simulink model "voxel_cloud_node_debag"  (R2021b)
settings: Solver=FixedStepAuto  StartTime=0.0  StopTime=10.0  RelTol=1e-3
model workspace (MAT data in the model file):
  Logfile_Data_Object = ros2bag
  Logfile_Data_Object.FilePath = 'C:\Users\takumi onozawa\Documents\MATLAB\ros2bag\lidars_point_raw_0.db3'
  Logfile_Data_Object.StartTime = 1633675920681641206
  Logfile_Data_Object.EndTime = 1633676017682751873
  Logfile_Data_Object.AvailableTopics = table
  Logfile_Data_Object.AvailableTopics.data{1} = [969; 970]
  Logfile_Data_Object.AvailableTopics.data{2} = categorical
  Logfile_Data_Object.AvailableTopics.data{2}.categoryNames = {'sensor_msgs/PointCloud2'}
  Logfile_Data_Object.AvailableTopics.data{2}.codes = [1; 1]
  Logfile_Data_Object.AvailableTopics.data{3}{1} = '% contain additional information such as normals, intensity, etc. The
    | % point data is stored as a binary blob, its layout described by the
    | % contents of the "fields" array.
    | %
    | % The point cloud data may be organized 2d (image-like) or 1d (unordered).
    | % Point clouds organized as 2d images may be produced by camera depth sensors
    | % such as stereo or Time-of-flight.
    | 
    | % Time of sensor data acquisition, and the coordinate frame ID (for 3d points).
    | std_msgs/Header header
    | 
    | % 2D structure of the point cloud. If the cloud is unordered, height is
    | % 1 and width is the length of the point cloud.
    | uint32 height
    | uint32 width
    | 
    | % Describes the channels and their layout in the binary data blob.
    | PointField[] fields
    | 
    | logical    is_bigendian % Is this data bigendian?
    | uint32  point_step      % Length of a point in bytes
    | uint32  row_step        % Length of a row in bytes
    | uint8[] data            % Actual point data, size is (row_step*height)
    | 
    | logical is_dense        % True if there are no invalid points'
  Logfile_Data_Object.AvailableTopics.data{3}{2} = '% contain additional information such as normals, intensity, etc. The
    | % point data is stored as a binary blob, its layout described by the
    | % contents of the "fields" array.
    | %
    | % The point cloud data may be organized 2d (image-like) or 1d (unordered).
    | % Point clouds organized as 2d images may be produced by camera depth sensors
    | % such as stereo or Time-of-flight.
    | 
    | % Time of sensor data acquisition, and the coordinate frame ID (for 3d points).
    | std_msgs/Header header
    | 
    | % 2D structure of the point cloud. If the cloud is unordered, height is
    | % 1 and width is the length of the point cloud.
    | uint32 height
    | uint32 width
    | 
    | % Describes the channels and their layout in the binary data blob.
    | PointField[] fields
    | 
    | logical    is_bigendian % Is this data bigendian?
    | uint32  point_step      % Length of a point in bytes
    | uint32  row_step        % Length of a row in bytes
    | uint8[] data            % Actual point data, size is (row_step*height)
    | 
    | logical is_dense        % True if there are no invalid points'
  Logfile_Data_Object.AvailableTopics.ndims = 2
  Logfile_Data_Object.AvailableTopics.nrows = 2
  Logfile_Data_Object.AvailableTopics.rownames = {'/lidar_front/points_raw'; '/lidar_rear/points_raw'}
  Logfile_Data_Object.AvailableTopics.nvars = 3
  Logfile_Data_Object.AvailableTopics.varnames = {'NumMessages', 'MessageType', 'MessageDefinition'}
  Logfile_Data_Object.AvailableTopics.props.useVariableNamesOriginal = 0
  Logfile_Data_Object.AvailableTopics.props.useDimensionNamesOriginal = 0
  Logfile_Data_Object.AvailableTopics.props.CustomProps = struct()
  Logfile_Data_Object.AvailableTopics.props.VariableCustomProps = struct()
  Logfile_Data_Object.AvailableTopics.props.versionSavedFrom = 4
  Logfile_Data_Object.AvailableTopics.props.minCompatibleVersion = 1
  Logfile_Data_Object.AvailableTopics.props.incompatibilityMsg = ''
  Logfile_Data_Object.AvailableTopics.props.VersionSavedFrom = 4
  Logfile_Data_Object.AvailableTopics.props.Description = ''
  Logfile_Data_Object.AvailableTopics.props.VariableNamesOriginal = {}
  Logfile_Data_Object.AvailableTopics.props.DimensionNames = {'Row', 'Variables'}
  Logfile_Data_Object.AvailableTopics.props.DimensionNamesOriginal = {}
  Logfile_Data_Object.AvailableTopics.props.UserData = []
  Logfile_Data_Object.AvailableTopics.props.VariableDescriptions = {}
  Logfile_Data_Object.AvailableTopics.props.VariableUnits = {}
  Logfile_Data_Object.AvailableTopics.props.VariableContinuity = {}
  Logfile_Data_Object.MessageList = table
  Logfile_Data_Object.MessageList.data{1} = [1633675920681641206 1633675920704850047 1633675920710280571 1633675920841302537 1633675920849007917 1633675920944718285 1633675920950454411 1633675921046456357 1633675921051238695 1633675921143527086 1633675921154682295 1633675921262758351 ... (1939 elements, 1939x1)]
  Logfile_Data_Object.MessageList.data{2} = categorical
  Logfile_Data_Object.MessageList.data{2}.categoryNames = {'/lidar_rear/points_raw'; '/lidar_front/points_raw'}
  Logfile_Data_Object.MessageList.data{2}.codes = [1 2 1 2 1 2 1 2 1 2 1 2 ... (1939 elements, 1939x1)]
  Logfile_Data_Object.MessageList.data{3} = categorical
  Logfile_Data_Object.MessageList.data{3}.categoryNames = {'sensor_msgs/PointCloud2'}
  Logfile_Data_Object.MessageList.data{3}.codes = [1 1 1 1 1 1 1 1 1 1 1 1 ... (1939 elements, 1939x1)]
  Logfile_Data_Object.MessageList.ndims = 2
  Logfile_Data_Object.MessageList.nrows = 1939
  Logfile_Data_Object.MessageList.nvars = 3
  Logfile_Data_Object.MessageList.varnames = {'Time', 'Topic', 'MessageType'}
  Logfile_Data_Object.MessageList.props.useVariableNamesOriginal = 0
  Logfile_Data_Object.MessageList.props.useDimensionNamesOriginal = 0
  Logfile_Data_Object.MessageList.props.CustomProps = struct()
  Logfile_Data_Object.MessageList.props.VariableCustomProps = struct()
  Logfile_Data_Object.MessageList.props.versionSavedFrom = 4
  Logfile_Data_Object.MessageList.props.minCompatibleVersion = 1
  Logfile_Data_Object.MessageList.props.incompatibilityMsg = ''
  Logfile_Data_Object.MessageList.props.VersionSavedFrom = 4
  Logfile_Data_Object.MessageList.props.Description = ''
  Logfile_Data_Object.MessageList.props.VariableNamesOriginal = {}
  Logfile_Data_Object.MessageList.props.DimensionNames = {'Row', 'Variables'}
  Logfile_Data_Object.MessageList.props.DimensionNamesOriginal = {}
  Logfile_Data_Object.MessageList.props.UserData = []
  Logfile_Data_Object.MessageList.props.VariableDescriptions = {}
  Logfile_Data_Object.MessageList.props.VariableUnits = {}
  Logfile_Data_Object.MessageList.props.VariableContinuity = {}
  Logfile_Data_Object.TopicTypeMap = containers.Map
  Logfile_Data_Object.TopicTypeMap.serialization.keys = {'/lidar_front/points_raw', '/lidar_rear/points_raw'}
  Logfile_Data_Object.TopicTypeMap.serialization.values = {'sensor_msgs/PointCloud2', 'sensor_msgs/PointCloud2'}
  Logfile_Data_Object.TopicTypeMap.serialization.uniformity = 1
  Logfile_Data_Object.TopicTypeMap.serialization.keyType = 'char'
  Logfile_Data_Object.TopicTypeMap.serialization.valueType = 'char'
  Logfile_Data_Object.TopicDefinitionMap = containers.Map
  Logfile_Data_Object.TopicDefinitionMap.serialization.keys = {'/lidar_front/points_raw', '/lidar_rear/points_raw'}
  Logfile_Data_Object.TopicDefinitionMap.serialization.values{1} = '% contain additional information such as normals, intensity, etc. The
    | % point data is stored as a binary blob, its layout described by the
    | % contents of the "fields" array.
    | %
    | % The point cloud data may be organized 2d (image-like) or 1d (unordered).
    | % Point clouds organized as 2d images may be produced by camera depth sensors
    | % such as stereo or Time-of-flight.
    | 
    | % Time of sensor data acquisition, and the coordinate frame ID (for 3d points).
    | std_msgs/Header header
    | 
    | % 2D structure of the point cloud. If the cloud is unordered, height is
    | % 1 and width is the length of the point cloud.
    | uint32 height
    | uint32 width
    | 
    | % Describes the channels and their layout in the binary data blob.
    | PointField[] fields
    | 
    | logical    is_bigendian % Is this data bigendian?
    | uint32  point_step      % Length of a point in bytes
    | uint32  row_step        % Length of a row in bytes
    | uint8[] data            % Actual point data, size is (row_step*height)
    | 
    | logical is_dense        % True if there are no invalid points'
  Logfile_Data_Object.TopicDefinitionMap.serialization.values{2} = '% contain additional information such as normals, intensity, etc. The
    | % point data is stored as a binary blob, its layout described by the
    | % contents of the "fields" array.
    | %
    | % The point cloud data may be organized 2d (image-like) or 1d (unordered).
    | % Point clouds organized as 2d images may be produced by camera depth sensors
    | % such as stereo or Time-of-flight.
    | 
    | % Time of sensor data acquisition, and the coordinate frame ID (for 3d points).
    | std_msgs/Header header
    | 
    | % 2D structure of the point cloud. If the cloud is unordered, height is
    | % 1 and width is the length of the point cloud.
    | uint32 height
    | uint32 width
    | 
    | % Describes the channels and their layout in the binary data blob.
    | PointField[] fields
    | 
    | logical    is_bigendian % Is this data bigendian?
    | uint32  point_step      % Length of a point in bytes
    | uint32  row_step        % Length of a row in bytes
    | uint8[] data            % Actual point data, size is (row_step*height)
    | 
    | logical is_dense        % True if there are no invalid points'
  Logfile_Data_Object.TopicDefinitionMap.serialization.uniformity = 1
  Logfile_Data_Object.TopicDefinitionMap.serialization.keyType = 'char'
  Logfile_Data_Object.TopicDefinitionMap.serialization.valueType = 'char'
  Logfile_Path = 'C:\Users\takumi onozawa\Documents\MATLAB\ros2bag\lidars_point_raw_0.db3'
  Logfile_Playback_Duration = nan
  Logfile_Playback_Offset = nan
  SL_ROS_VariableLengthArrays_MaxSizes.CommonInfo.ArrayTruncateAction = 'EmitWarning'
  SL_ROS_VariableLengthArrays_MaxSizes.MsgTypeMap = containers.Map
  SL_ROS_VariableLengthArrays_MaxSizes.MsgTypeMap.serialization.keys = {'sensor_msgs/PointCloud2'}
  SL_ROS_VariableLengthArrays_MaxSizes.MsgTypeMap.serialization.values{1}(1).PropertyName = 'data'
  SL_ROS_VariableLengthArrays_MaxSizes.MsgTypeMap.serialization.values{1}(1).DataType = 'uint8'
  SL_ROS_VariableLengthArrays_MaxSizes.MsgTypeMap.serialization.values{1}(1).MaxLength = 1760000
  SL_ROS_VariableLengthArrays_MaxSizes.MsgTypeMap.serialization.values{1}(2).PropertyName = 'fields'
  SL_ROS_VariableLengthArrays_MaxSizes.MsgTypeMap.serialization.values{1}(2).DataType = 'sensor_msgs/PointField'
  SL_ROS_VariableLengthArrays_MaxSizes.MsgTypeMap.serialization.values{1}(2).MaxLength = 16
  SL_ROS_VariableLengthArrays_MaxSizes.MsgTypeMap.serialization.uniformity = 0
  SL_ROS_VariableLengthArrays_MaxSizes.MsgTypeMap.serialization.keyType = 'char'
  SL_ROS_VariableLengthArrays_MaxSizes.MsgTypeMap.serialization.valueType = 'any'
undefined symbols (not defined in the file or in its folder): height, row_step, width
libraries: ros2lib x4, simulink x4
settings Model: Creator=takum  LastModifiedBy=takumi onozawa
settings SolverCC: AlgebraicLoopSolver=TrustRegion
settings OptimizationCC: EnhancedBackFolding=on  PassReuseOutputArgsAs=Individual arguments  ZeroExternalMemoryAtStartup=off  ZeroInternalMemoryAtStartup=off  MaxStackSize=64  OptimizeBlockOrder=speed  DifferentSizesBufferReuse=on  OptimizationCustomize=off  EfficientTunableParamExpr=on
settings DebuggingCC: ParameterTunabilityLossMsg=error  SFMachineParentedDataDiag=warning
settings SFSimCC: MATLABDynamicMemAlloc=off
settings RTWCC: Description=Embedded Coder  SystemTargetFile=ert.tlc  HardwareBoard=Robot Operating System 2 (ROS 2)  TemplateMakefile=ert_default_tmf  Toolchain=Colcon Tools  TargetLang=C++
settings CodeAppCC: ForceParamTrailComments=on  IgnoreCustomStorageClasses=off  OperatorAnnotations=on  SimulinkDataObjDesc=on  SFDataObjDesc=on  InsertBlockDesc=on
settings ERTTargetCC: CodeInterfacePackaging=C++ class  RootIOFormat=Structure reference

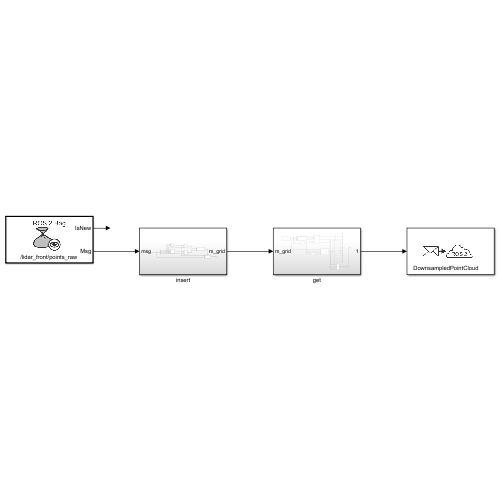
[thumbnail: Simulink's stored preview of the top-level diagram]
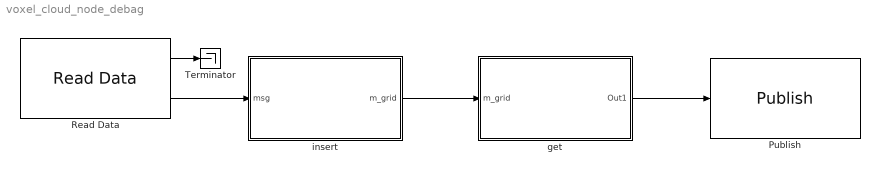
== system voxel_cloud_node_debag ==
  Publish : ros2lib/Publish  topicSource=Specify your own  topic=DownsampledPointCloud  messageType=sensor_msgs/PointCloud2  QOSHistory=Keep last  QOSDepth=1  QOSReliability=Reliable  QOSDurability=Volatile
      settings: SourceProductBaseCode=RR
  Read Data : ros2lib/Read Data  topic=/lidar_front/points_raw  sampleTime=-1  logfileType=rosbag2  modelName=voxel_cloud_node_debag  msgType=sensor_msgs/PointCloud2
      settings: SourceProductBaseCode=RR
  Terminator : Terminator
  get : Subsystem
  insert : Subsystem
  wires:
  Read Data/1 -> Terminator/1
  Read Data/2 -> insert/1(msg)
  get/1(Out1) -> Publish/1
  insert/1(m_grid) -> get/1(m_grid)

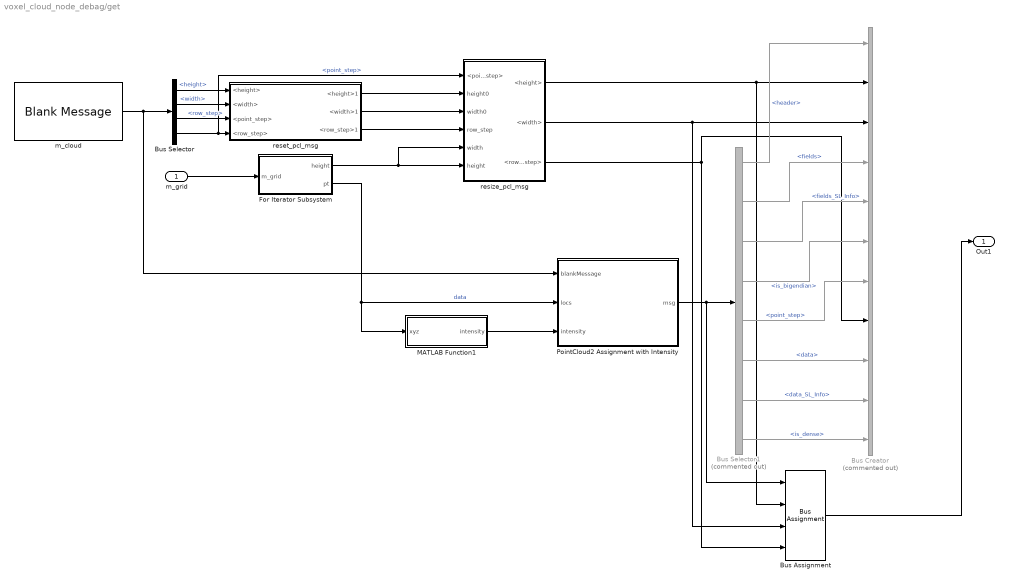
== system voxel_cloud_node_debag/get ==
  m_grid : Inport
  Bus Assignment : BusAssignment  AssignedSignals=height,width,row_step
  Bus Creator : BusCreator  Commented=on  Inputs=11
  Bus Selector : BusSelector  OutputSignals=height,width,row_step,point_step
  Bus Selector1 : BusSelector  Commented=on  OutputSignals=header,fields,fields_SL_Info,is_bigendian,point_step,data,data_SL_Info,is_dense
  For Iterator Subsystem : Subsystem  TreatAsAtomicUnit=on
  MATLAB Function1 : MATLAB Function  TreatAsAtomicUnit=on
  PointCloud2 Assignment with Intensity : MATLAB Function  TreatAsAtomicUnit=on
  m_cloud : ros2lib/Blank Message  messageClass=Message  entityType=sensor_msgs/PointCloud2  messageType=sensor_msgs/PointCloud2  SampleTime=inf
      settings: SourceProductBaseCode=RR
  reset_pcl_msg : Subsystem
  resize_pcl_msg : Subsystem
  Out1 : Outport
  wires:
  m_grid/1 -> For Iterator Subsystem/1(m_grid)
  Bus Selector/2 -> reset_pcl_msg/2(<width>)  "<width>"
  Bus Selector/3 -> reset_pcl_msg/3(<point_step>)  "<row_step>"
  Bus Selector/1 -> reset_pcl_msg/1(<height>)  "<height>"
  For Iterator Subsystem/2(pt) -> PointCloud2 Assignment with Intensity/2(locs), MATLAB Function1/1(xyz)  "data"
  Bus Selector/4 -> resize_pcl_msg/1(<point_step>), reset_pcl_msg/4(<row_step>)  "<point_step>"
  resize_pcl_msg/3(<row_step>) -> Bus Creator/8, Bus Assignment/4
  resize_pcl_msg/2(<width>) -> Bus Assignment/3, Bus Creator/3
  reset_pcl_msg/1(<height>1) -> resize_pcl_msg/2(height0)
  reset_pcl_msg/3(<row_step>1) -> resize_pcl_msg/4(row_step)
  reset_pcl_msg/2(<width>1) -> resize_pcl_msg/3(width0)
  resize_pcl_msg/1(<height>) -> Bus Assignment/2, Bus Creator/2
  For Iterator Subsystem/1(height) -> resize_pcl_msg/5(width), resize_pcl_msg/6(height)
  Bus Assignment/1 -> Out1/1
  PointCloud2 Assignment with Intensity/1(msg) -> Bus Assignment/1, Bus Selector1/1
  m_cloud/1 -> PointCloud2 Assignment with Intensity/1(blankMessage), Bus Selector/1
  Bus Selector1/1 -> Bus Creator/1  "<header>"
  Bus Selector1/2 -> Bus Creator/4  "<fields>"
  Bus Selector1/3 -> Bus Creator/5  "<fields_SL_Info>"
  Bus Selector1/4 -> Bus Creator/6  "<is_bigendian>"
  Bus Selector1/5 -> Bus Creator/7  "<point_step>"
  Bus Selector1/6 -> Bus Creator/9  "<data>"
  Bus Selector1/7 -> Bus Creator/10  "<data_SL_Info>"
  Bus Selector1/8 -> Bus Creator/11  "<is_dense>"
  MATLAB Function1/1(intensity) -> PointCloud2 Assignment with Intensity/3(intensity)

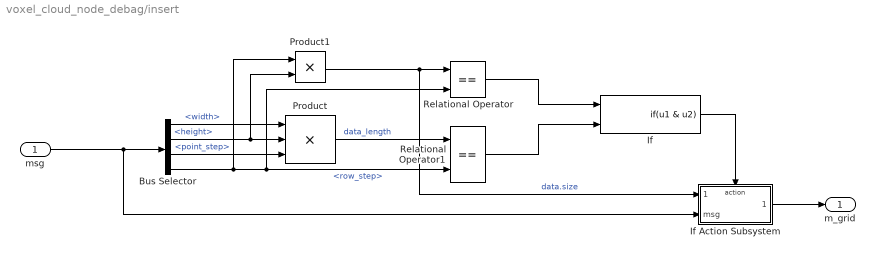
== system voxel_cloud_node_debag/insert ==
  msg : Inport
  Bus Selector : BusSelector  OutputSignals=width,height,point_step,row_step
  If : If  NumInputs=2  IfExpression=u1 & u2  ShowElse=off
  If Action Subsystem : Subsystem  TreatAsAtomicUnit=on
  Product : Product  Inputs=3
  Product1 : Product  OutDataTypeStr=uint32
  Relational Operator : RelationalOperator  Operator===  OutDataTypeStr=boolean  RndMeth=Simplest
  Relational Operator1 : RelationalOperator  Operator===  OutDataTypeStr=boolean  RndMeth=Simplest
  m_grid : Outport
  wires:
  If Action Subsystem/1(m_grid) -> m_grid/1
  Bus Selector/1 -> Product/1  "<width>"
  Bus Selector/2 -> Product/2, Product1/2  "<height>"
  Bus Selector/3 -> Product/3  "<point_step>"
  Product/1 -> Relational Operator1/1  "data_length"
  Bus Selector/4 -> Relational Operator1/2, Relational Operator/2, Product1/1  "<row_step>"
  Product1/1 -> If Action Subsystem/1(data.size), Relational Operator/1  "data.size"
  Relational Operator/1 -> If/1
  Relational Operator1/1 -> If/2
  If/1 -> If Action Subsystem/Action
  msg/1 -> Bus Selector/1, If Action Subsystem/2(msg)

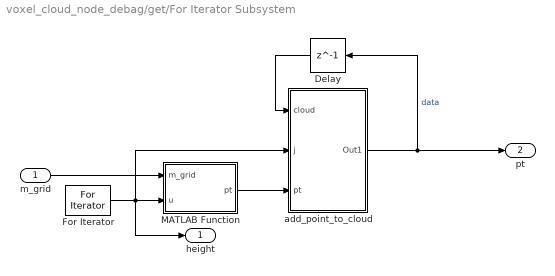
== system voxel_cloud_node_debag/get/For Iterator Subsystem ==
  m_grid : Inport
  Delay : Delay  DelayLength=1
  For Iterator : ForIterator  IterationLimit=55000
  MATLAB Function : MATLAB Function  TreatAsAtomicUnit=on
  add_point_to_cloud : Subsystem
  height : Outport
  pt : Outport  Port=2
  wires:
  m_grid/1 -> MATLAB Function/1(m_grid)
  MATLAB Function/1(pt) -> add_point_to_cloud/3(pt)
  For Iterator/1 -> height/1, add_point_to_cloud/2(j), MATLAB Function/2(u)
  add_point_to_cloud/1(Out1) -> Delay/1, pt/1  "data"
  Delay/1 -> add_point_to_cloud/1(cloud)

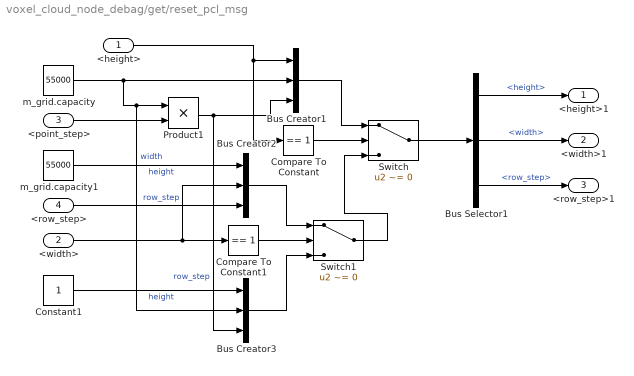
== system voxel_cloud_node_debag/get/reset_pcl_msg ==
  <height> : Inport
  <width> : Inport  Port=2
  <point_step> : Inport  Port=3
  <row_step> : Inport  Port=4
  Bus Creator1 : BusCreator  Inputs=3
  Bus Creator2 : BusCreator  Inputs=3
  Bus Creator3 : BusCreator  Inputs=3
  Bus Selector1 : BusSelector  OutputSignals=height,width,row_step
  Compare To Constant : simulink/Logic and Bit Operations/Compare To Constant  relop===  const=1  OutDataTypeStr=boolean
  Compare To Constant1 : simulink/Logic and Bit Operations/Compare To Constant  relop===  const=1  OutDataTypeStr=boolean
  Constant1 : Constant  OutDataTypeStr=uint32
  Product1 : Product  OutDataTypeStr=uint32
  Switch : Switch  Criteria=u2 ~= 0
  Switch1 : Switch  Criteria=u2 ~= 0
  m_grid.capacity : Constant  Value=55000  OutDataTypeStr=uint32
  m_grid.capacity1 : Constant  Value=55000  OutDataTypeStr=uint32
  <height>1 : Outport
  <width>1 : Outport  Port=2
  <row_step>1 : Outport  Port=3
  wires:
  <point_step>/1 -> Product1/2
  m_grid.capacity/1 -> Product1/1, Bus Creator3/2, Bus Creator1/2  "width"
  Switch/1 -> Bus Selector1/1
  Product1/1 -> Bus Creator1/3, Bus Creator3/3  "row_step"
  m_grid.capacity1/1 -> Bus Creator2/1  "height"
  Bus Creator2/1 -> Switch1/1
  Bus Creator1/1 -> Switch/1
  <height>/1 -> Compare To Constant/1, Bus Creator1/1
  Constant1/1 -> Bus Creator3/1  "height"
  Bus Creator3/1 -> Switch1/3
  Compare To Constant1/1 -> Switch1/2
  Switch1/1 -> Switch/3
  <width>/1 -> Bus Creator2/2, Compare To Constant1/1
  Compare To Constant/1 -> Switch/2
  Bus Selector1/1 -> <height>1/1  "<height>"
  <row_step>/1 -> Bus Creator2/3  "row_step"
  Bus Selector1/2 -> <width>1/1  "<width>"
  Bus Selector1/3 -> <row_step>1/1  "<row_step>"

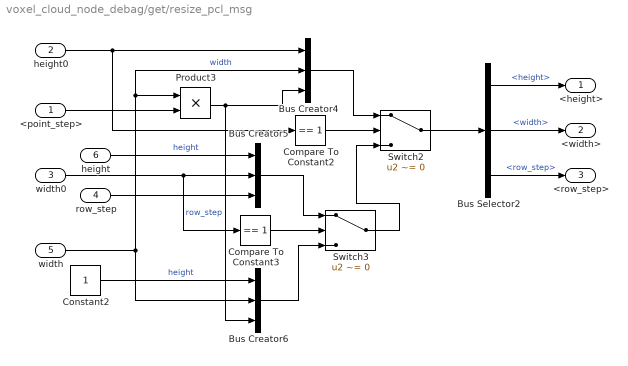
== system voxel_cloud_node_debag/get/resize_pcl_msg ==
  <point_step> : Inport
  height0 : Inport  Port=2
  width0 : Inport  Port=3
  row_step : Inport  Port=4
  width : Inport  Port=5
  height : Inport  Port=6
  Bus Creator4 : BusCreator  Inputs=3
  Bus Creator5 : BusCreator  Inputs=3
  Bus Creator6 : BusCreator  Inputs=3
  Bus Selector2 : BusSelector  OutputSignals=height,width,row_step
  Compare To Constant2 : simulink/Logic and Bit Operations/Compare To Constant  relop===  const=1  OutDataTypeStr=boolean
  Compare To Constant3 : simulink/Logic and Bit Operations/Compare To Constant  relop===  const=1  OutDataTypeStr=boolean
  Constant2 : Constant  OutDataTypeStr=uint32
  Product3 : Product  OutDataTypeStr=uint32
  Switch2 : Switch  Criteria=u2 ~= 0
  Switch3 : Switch  Criteria=u2 ~= 0
  <height> : Outport
  <width> : Outport  Port=2
  <row_step> : Outport  Port=3
  wires:
  Compare To Constant3/1 -> Switch3/2
  Bus Creator6/1 -> Switch3/3
  Switch2/1 -> Bus Selector2/1
  Product3/1 -> Bus Creator4/3, Bus Creator6/3  "row_step"
  Switch3/1 -> Switch2/3
  Bus Selector2/1 -> <height>/1  "<height>"
  width/1 -> Bus Creator6/2, Bus Creator4/2, Product3/1  "width"
  Bus Creator5/1 -> Switch3/1
  Constant2/1 -> Bus Creator6/1  "height"
  Bus Creator4/1 -> Switch2/1
  Compare To Constant2/1 -> Switch2/2
  height0/1 -> Compare To Constant2/1, Bus Creator4/1
  width0/1 -> Compare To Constant3/1, Bus Creator5/2
  Bus Selector2/3 -> <row_step>/1  "<row_step>"
  <point_step>/1 -> Product3/2
  row_step/1 -> Bus Creator5/3
  Bus Selector2/2 -> <width>/1  "<width>"
  height/1 -> Bus Creator5/1  "height"

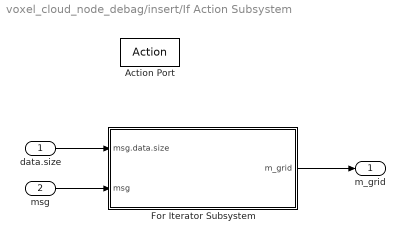
== system voxel_cloud_node_debag/insert/If Action Subsystem ==
  data.size : Inport
  msg : Inport  Port=2
  Action Port : ActionPort  ActionPortLabel=if(u1 & u2)
  For Iterator Subsystem : Subsystem  TreatAsAtomicUnit=on
  m_grid : Outport
  wires:
  data.size/1 -> For Iterator Subsystem/1(msg.data.size)
  msg/1 -> For Iterator Subsystem/2(msg)
  For Iterator Subsystem/1(m_grid) -> m_grid/1

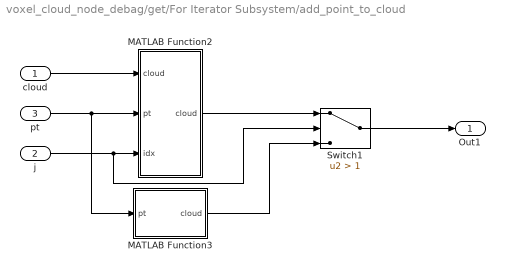
== system voxel_cloud_node_debag/get/For Iterator Subsystem/add_point_to_cloud ==
  cloud : Inport
  j : Inport  Port=2
  pt : Inport  Port=3
  MATLAB Function2 : MATLAB Function  TreatAsAtomicUnit=on
  MATLAB Function3 : MATLAB Function  TreatAsAtomicUnit=on
  Switch1 : Switch  Criteria=u2 > Threshold  Threshold=1
  Out1 : Outport
  wires:
  MATLAB Function2/1(cloud) -> Switch1/1
  pt/1 -> MATLAB Function3/1(pt), MATLAB Function2/2(pt)
  j/1 -> Switch1/2, MATLAB Function2/3(idx)
  Switch1/1 -> Out1/1
  MATLAB Function3/1(cloud) -> Switch1/3
  cloud/1 -> MATLAB Function2/1("cloud ")

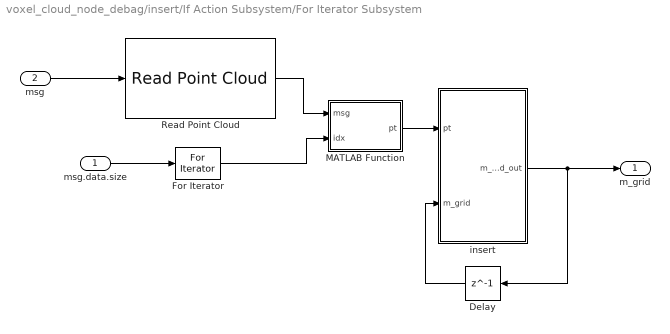
== system voxel_cloud_node_debag/insert/If Action Subsystem/For Iterator Subsystem ==
  msg.data.size : Inport
  msg : Inport  Port=2
  Delay : Delay  DelayLength=1
  For Iterator : ForIterator  IterationSource=external
  MATLAB Function : MATLAB Function  TreatAsAtomicUnit=on
  Read Point Cloud : ros2lib/Read Point Cloud  MaximumPointCloudSize=[480, 640]  PreserveStructure=off  ShowRGBOutput=off  ShowIntensityOutput=off  ShowErrorCodeOutput=off  VariableSizeOutputs=off
      settings: SourceProductBaseCode=RR
  insert : Subsystem
  m_grid : Outport
  wires:
  msg/1 -> Read Point Cloud/1
  msg.data.size/1 -> For Iterator/1
  insert/1(m_grid_out) -> Delay/1, m_grid/1
  Delay/1 -> insert/2(m_grid)
  For Iterator/1 -> MATLAB Function/2(idx)
  MATLAB Function/1(pt) -> insert/1(pt)
  Read Point Cloud/1 -> MATLAB Function/1(msg)

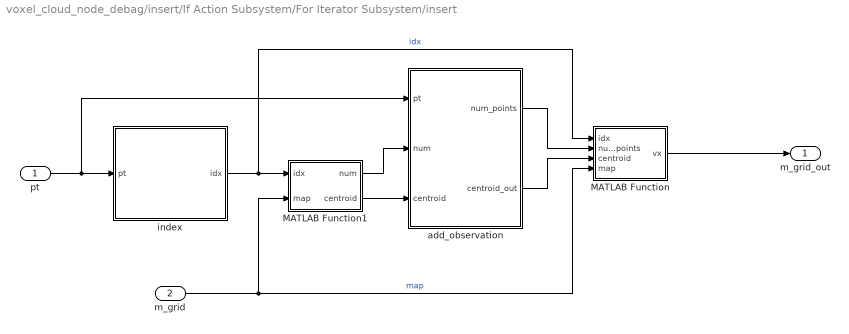
== system voxel_cloud_node_debag/insert/If Action Subsystem/For Iterator Subsystem/insert ==
  pt : Inport
  m_grid : Inport  Port=2
  MATLAB Function : MATLAB Function  TreatAsAtomicUnit=on
  MATLAB Function1 : MATLAB Function  TreatAsAtomicUnit=on
  add_observation : Subsystem
  index : Subsystem
  m_grid_out : Outport
  wires:
  pt/1 -> add_observation/1(pt), index/1(pt)
  index/1(idx) -> MATLAB Function/1(idx), MATLAB Function1/1(idx)  "idx"
  m_grid/1 -> MATLAB Function/4(map), MATLAB Function1/2(map)  "map"
  MATLAB Function/1(vx) -> m_grid_out/1
  MATLAB Function1/1(num) -> add_observation/2(num)
  add_observation/1(num_points) -> MATLAB Function/2(num_points)
  add_observation/2(centroid_out) -> MATLAB Function/3(centroid)
  MATLAB Function1/2(centroid) -> add_observation/3(centroid)

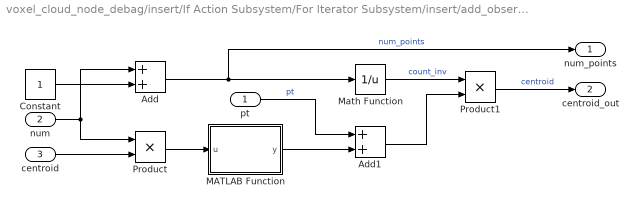
== system voxel_cloud_node_debag/insert/If Action Subsystem/For Iterator Subsystem/insert/add_observation ==
  pt : Inport
  num : Inport  Port=2
  centroid : Inport  Port=3
  Add : Sum  OutDataTypeStr=uint32
  Add1 : Sum
  Constant : Constant
  MATLAB Function : MATLAB Function  TreatAsAtomicUnit=on
  Math Function : Math  Operator=reciprocal  SaturateOnIntegerOverflow=on
  Product : Product  OutDataTypeStr=uint32
  Product1 : Product  OutDataTypeStr=double
  num_points : Outport
  centroid_out : Outport  Port=2
  wires:
  num/1 -> Product/1, Add/1
  Add/1 -> num_points/1, Math Function/1  "num_points"
  Math Function/1 -> Product1/1  "count_inv"
  Add1/1 -> Product1/2
  Product1/1 -> centroid_out/1  "centroid"
  Constant/1 -> Add/2
  Product/1 -> MATLAB Function/1(u)
  centroid/1 -> Product/2
  pt/1 -> Add1/1  "pt"
  MATLAB Function/1(y) -> Add1/2

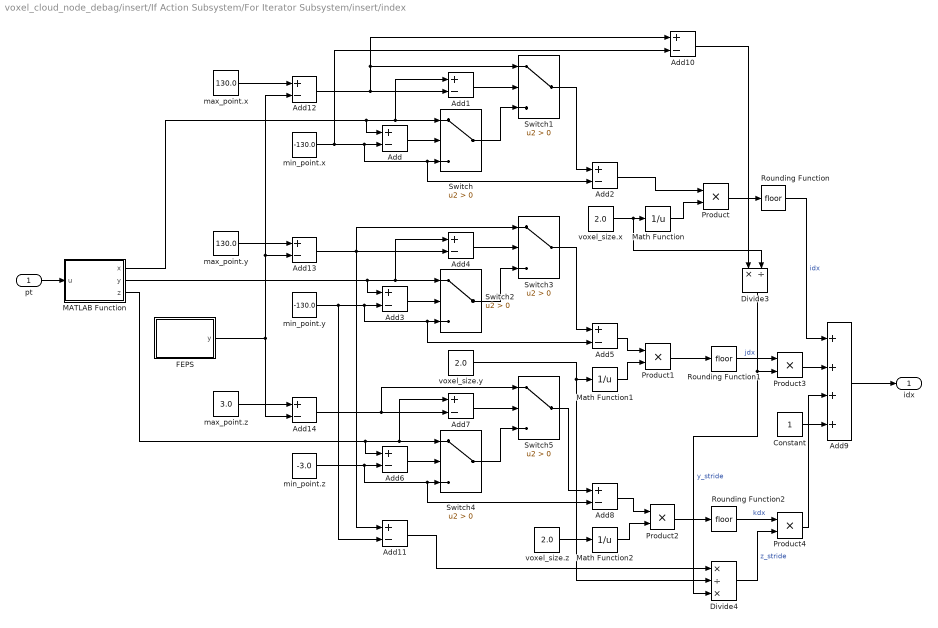
== system voxel_cloud_node_debag/insert/If Action Subsystem/For Iterator Subsystem/insert/index ==
  pt : Inport
  Add{,1..8,10..14} (14 alike) : Sum  Inputs=+-
  Add9 : Sum  Inputs=4  OutDataTypeStr=uint32
  Constant : Constant
  Divide3 : Product  Inputs=*/
  Divide4 : Product  Inputs=*/*
  FEPS : MATLAB Function  TreatAsAtomicUnit=on
  MATLAB Function : MATLAB Function  TreatAsAtomicUnit=on
  Math Function : Math  Operator=reciprocal  SaturateOnIntegerOverflow=on
  Math Function1 : Math  Operator=reciprocal  SaturateOnIntegerOverflow=on
  Math Function2 : Math  Operator=reciprocal  SaturateOnIntegerOverflow=on
  Product{,1..4} (5 alike) : Product
  Rounding Function : Rounding
  Rounding Function1 : Rounding
  Rounding Function2 : Rounding
  Switch{,1..5} (6 alike) : Switch  Criteria=u2 > Threshold
  max_point.x : Constant  Value=130.0
  max_point.y : Constant  Value=130.0
  max_point.z : Constant  Value=3.0
  min_point.x : Constant  Value=-130.0
  min_point.y : Constant  Value=-130.0
  min_point.z : Constant  Value=-3.0
  voxel_size.x : Constant  Value=2.0
  voxel_size.y : Constant  Value=2.0
  voxel_size.z : Constant  Value=2.0
  idx : Outport
  wires:
  pt/1 -> MATLAB Function/1(u)
  Add13/1 -> Switch3/1, Add4/2, Add11/1
  Math Function/1 -> Product/2
  Switch1/1 -> Add2/1
  min_point.z/1 -> Add8/2, Switch4/3, Add6/2
  Product3/1 -> Add9/2
  min_point.y/1 -> Add5/2, Switch2/3, Add3/2, Add11/2
  voxel_size.z/1 -> Math Function2/1
  Add4/1 -> Switch3/2
  Divide4/1 -> Product4/2  "z_stride"
  voxel_size.y/1 -> Math Function1/1, Divide4/2
  FEPS/1(y) -> Add14/2, Add13/2, Add12/2
  voxel_size.x/1 -> Math Function/1, Divide3/2
  Add10/1 -> Divide3/1
  Add8/1 -> Product2/1
  Product2/1 -> Rounding Function2/1
  min_point.x/1 -> Add10/2, Add2/2, Switch/3, Add/2
  Add6/1 -> Switch4/2
  Add11/1 -> Divide4/1
  Add1/1 -> Switch1/2
  Product1/1 -> Rounding Function1/1
  Divide3/1 -> Divide4/3, Product3/2  "y_stride"
  Switch4/1 -> Switch5/3
  Switch3/1 -> Add5/1
  Product/1 -> Rounding Function/1
  Switch/1 -> Switch1/3
  Add/1 -> Switch/2
  Add14/1 -> Switch5/1, Add7/2
  Add5/1 -> Product1/1
  Add12/1 -> Add1/2, Add10/1, Switch1/1
  Switch2/1 -> Switch3/3
  Add3/1 -> Switch2/2
  Math Function1/1 -> Product1/2
  Add7/1 -> Switch5/2
  Product4/1 -> Add9/3
  Add2/1 -> Product/1
  Switch5/1 -> Add8/1
  max_point.x/1 -> Add12/1
  Math Function2/1 -> Product2/2
  max_point.y/1 -> Add13/1
  max_point.z/1 -> Add14/1
  Add9/1 -> idx/1
  MATLAB Function/2(y) -> Add3/1, Add4/1, Switch2/1
  MATLAB Function/1(x) -> Add/1, Add1/1, Switch/1
  MATLAB Function/3(z) -> Add6/1, Switch4/1, Add7/1
  Rounding Function/1 -> Add9/1  "idx"
  Rounding Function1/1 -> Product3/1  "jdx"
  Rounding Function2/1 -> Product4/1  "kdx"
  Constant/1 -> Add9/4

== matlab function voxel_cloud_node_debag/get/MATLAB Function1 ==
  data: xyz input; intensity output
function intensity = fcn(xyz)
intensity = rescale(xyz(:,3),0,255);

== matlab function voxel_cloud_node_debag/insert/If Action Subsystem/For Iterator Subsystem/MATLAB Function ==
  data: pt output; msg input; idx input
function pt = fcn(msg, idx)

pt = msg(idx,:);

== matlab function voxel_cloud_node_debag/insert/If Action Subsystem/For Iterator Subsystem/insert/MATLAB Function1 ==
  data: num output; idx input; map input; centroid output
function [num,centroid] = fcn(idx, map)

num = map(idx).num;
centroid = map(idx).centroid;

== matlab function voxel_cloud_node_debag/insert/If Action Subsystem/For Iterator Subsystem/insert/MATLAB Function ==
  data: idx input; num_points input; centroid input; map input; vx output Bus: BusObject size=55000,2
function vx = fcn(idx, num_points, centroid, map)

map(idx).num = num_points;
map(idx).centroid = permute(centroid,[2 1]);
vx = map;

== matlab function voxel_cloud_node_debag/get/For Iterator Subsystem/add_point_to_cloud/MATLAB Function2 ==
  data: cloud output size=[55000 3]; cloud input; pt input; idx input
function cloud = fcn(cloud,pt, idx)
cloud(idx,:) = pt;

== matlab function voxel_cloud_node_debag/get/For Iterator Subsystem/add_point_to_cloud/MATLAB Function3 ==
  data: cloud output; pt input
function cloud = fcn(pt)
cloud = zeros(55000,3);
cloud(1,:) = pt;

== matlab function voxel_cloud_node_debag/insert/If Action Subsystem/For Iterator Subsystem/insert/add_observation/MATLAB Function ==
  data: u input; y output
function y = fcn(u)

y = permute(u,[2 1]);

== matlab function voxel_cloud_node_debag/get/PointCloud2 Assignment with Intensity ==
  data: blankMessage input Bus: SL_Bus_sensor_msgs_PointCloud2; locs input; msg output Bus: SL_Bus_sensor_msgs_PointCloud2; intensity input
function msg = assignNestedArrayMessages(blankMessage,locs,intensity)
%#codegen

blankMessage.header.frame_id(1:3) = uint8('map');
blankMessage.header.frame_id_SL_Info.CurrentLength = uint32(3);
blankMessage.height = uint32(1);
blankMessage.width = uint32(size(locs,1));
blankMessage.point_step = uint32(32);
blankMessage.row_step = blankMessage.width * blankMessage.point_step;
blankMessage.fields_SL_Info.CurrentLength = uint32(4);
blankMessage.fields(1).name(1) = uint8('x');
blankMessage.fields(1).name_SL_Info.CurrentLength = uint32(1);
blankMessage.fields(1).offset = uint32(0);
blankMessage.fields(1).datatype = uint8(7);
blankMessage.fields(1).count = uint32(1);
blankMessage.fields(2).name(1) = uint8('y');
blankMessage.fields(2).name_SL_Info.CurrentLength = uint32(1);
blankMessage.fields(2).offset = uint32(4);
blankMessage.fields(2).datatype = uint8(7);
blankMessage.fields(2).count = uint32(1);
blankMessage.fields(3).name(1) = uint8('z');
blankMessage.fields(3).name_SL_Info.CurrentLength = uint32(1);
blankMessage.fields(3).offset = uint32(8);
blankMessage.fields(3).datatype = uint8(7);
blankMessage.fields(3).count = uint32(1);
blankMessage.fields(4).name(1:9) = uint8('intensity');
blankMessage.fields(4).name_SL_Info.CurrentLength = uint32(9);
blankMessage.fields(4).offset = uint32(16);
blankMessage.fields(4).datatype = uint8(7);
blankMessage.fields(4).count = uint32(1);

locs = reshape(locs,[],3);
intensity = reshape(intensity,[],1);
data = [locs zeros(size(locs,1),1,'single') intensity zeros(size(locs,1),3,'single')];
dataPacked = reshape(permute(data,[2 1]),[],1);
dataCasted = typecast(dataPacked,'uint8');
blankMessage.data(1:numel(dataCasted)) = dataCasted;
blankMessage.data_SL_Info.CurrentLength = uint32(numel(dataCasted));

msg = blankMessage;

== matlab function voxel_cloud_node_debag/insert/If Action Subsystem/For Iterator Subsystem/insert/index/MATLAB Function ==
  data: x output; u input; y output; z output
function [x,y,z] = fcn(u)

x = u(1);
y = u(2);
z = u(3);

== matlab function voxel_cloud_node_debag/insert/If Action Subsystem/For Iterator Subsystem/insert/index/FEPS ==
  data: y output
function y = fcn()

y = eps();

== matlab function voxel_cloud_node_debag/get/For Iterator Subsystem/MATLAB Function ==
  data: m_grid input; u input; pt output
function pt = fcn(m_grid, u)

pt = permute(m_grid(u).centroid,[2 1]);
